simulink model "Tachogenerator_sim_2020"  (R2020b)
settings: Solver=ode4  StartTime=0.0  StopTime=10.0  FixedStep=0.05  RelTol=1e-3
settings Model: Creator=005274  LastModifiedBy=005274

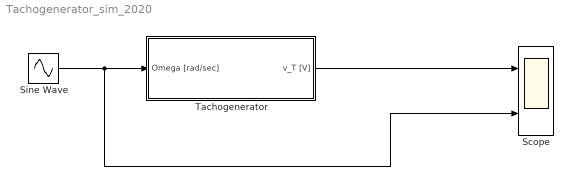
== system Tachogenerator_sim_2020 ==
  Scope : Scope  NumInputPorts=2
  Sine Wave : Sin  Amplitude=1000*2*pi/60  Frequency=2*pi  SampleTime=0
  Tachogenerator : Subsystem  mask(TachoGeneratorModel){}
  wires:
  Sine Wave/1 -> Scope/2, Tachogenerator/1(Omega [rad/sec])
  Tachogenerator/1(v_T [V]) -> Scope/1

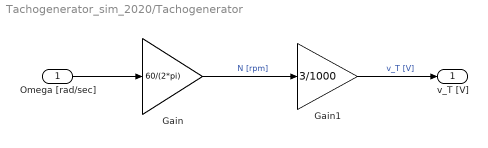
== system Tachogenerator_sim_2020/Tachogenerator ==
  Omega [rad/sec] : Inport
  Gain : Gain  Gain=60/(2*pi)
  Gain1 : Gain  Gain=3/1000
  v_T [V] : Outport
  wires:
  Gain/1 -> Gain1/1  "N [rpm]"
  Omega [rad/sec]/1 -> Gain/1
  Gain1/1 -> v_T [V]/1  "v_T [V]"
